simulink model "e01_simulink"  (R2023b)
settings: Solver=VariableStepAuto  StartTime=0.0  StopTime=25  RelTol=1e-3
values from neighbouring files (symbols this model uses):
  A_mat = double(A_mat)    [e01.m]
  B_mat = double(B_mat)    [e01.m]
  C_mat = double(C_mat)    [e01.m]
  D_mat = double(D_mat)    [e01.m]
  g = 9.81    [e01.m]
  Im0 = 0.8    [e01.m]
  Km = 1.52e-4    (= 0.000152)    [e01.m]
  Kt = 708.27    [e01.m]
  m = 0.02    [e01.m]
  X0 = [0.0223, 0]'    [e01.m]
  x1_eq = X0(1)    [e01.m]
settings Model: Creator=Marco  LastModifiedBy=Marco

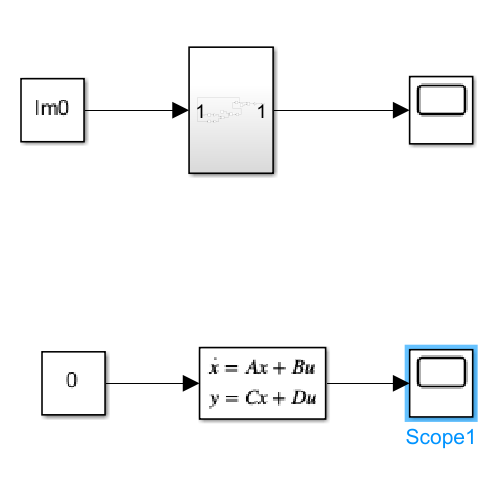
[thumbnail: Simulink's stored preview of the top-level diagram]
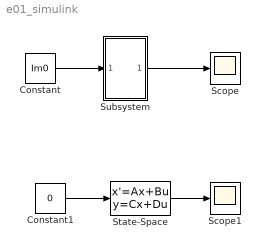
== system e01_simulink ==
  Constant : Constant  Value=Im0
  Constant1 : Constant  Value=0
  Scope : Scope
  Scope1 : Scope
  State-Space : StateSpace  A=A_mat  B=B_mat  C=C_mat  D=D_mat  InitialCondition=[0,0]'
  Subsystem : Subsystem
  wires:
  Constant/1 -> Subsystem/1(In1)
  Subsystem/1(Out1) -> Scope/1
  Constant1/1 -> State-Space/1
  State-Space/1 -> Scope1/1

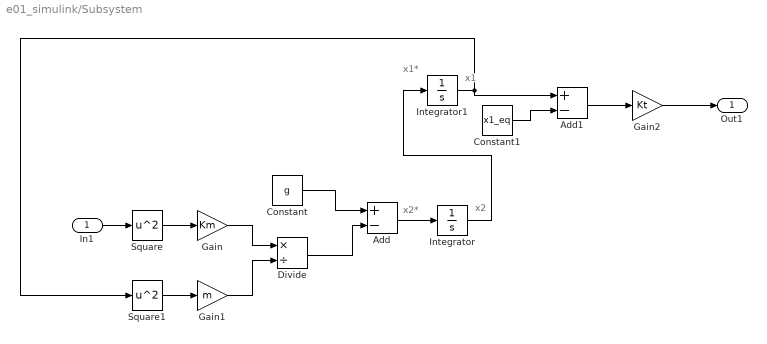
== system e01_simulink/Subsystem ==
  note: x1
  note: x2*
  note: x1*
  note: x2
  In1 : Inport
  Add : Sum  Inputs=+-
  Add1 : Sum  Inputs=+-
  Constant : Constant  Value=g
  Constant1 : Constant  Value=x1_eq
  Divide : Product  Inputs=*/
  Gain : Gain  Gain=Km
  Gain1 : Gain  Gain=m
  Gain2 : Gain  Gain=Kt
  Integrator : Integrator  InitialCondition=X0(2)
  Integrator1 : Integrator  InitialCondition=x1_eq
  Square : Math  Operator=square
  Square1 : Math  Operator=square
  Out1 : Outport
  wires:
  Constant/1 -> Add/1
  Add/1 -> Integrator/1
  Constant1/1 -> Add1/2
  Square1/1 -> Gain1/1
  Integrator/1 -> Integrator1/1
  Integrator1/1 -> Square1/1, Add1/1
  Divide/1 -> Add/2
  Add1/1 -> Gain2/1
  Square/1 -> Gain/1
  In1/1 -> Square/1
  Gain1/1 -> Divide/2
  Gain2/1 -> Out1/1
  Gain/1 -> Divide/1
